simulink model "Control_model_10DOF_fin"  (R2016b)
settings: Solver=FixedStepAuto  StartTime=0.0  StopTime=10  FixedStep=0.0001  RelTol=1e-3
InitFcn:
  | Initialisation_ctr_10DOF_fin
values from neighbouring files (symbols this model uses):
  COM_Parameters = [-lpelvis/2;r2;0]    [Initialisation_ctr_10DOF_fin.m]
  DH_Parameters = [hfoot 0 ... (first row only)    [Initialisation_ctr_10DOF_fin.m]
  dTrunk = trunklbd(3)    [Initialisation_ctr_10DOF_fin.m]
  dxFootSM = dxFoot    [Initialisation_ctr_10DOF_fin.m]
  dxTrunk = 0.1    [Initialisation_ctr_10DOF_fin.m]
  Foot_Parameters = [0;-(lFoot/2-lHeel);0]    [Initialisation_ctr_10DOF_fin.m]
  HAA2HEE = [0; 0; 0.001]    [Initialisation_ctr_10DOF_fin.m]
  HEE2HFE = 0.5*[0.2; 0; 0]    [Initialisation_ctr_10DOF_fin.m]
  height_vrp = CoM_position(1)    [Initialisation_ctr_10DOF_fin.m]
  hTrunk = trunklbd(1)    [Initialisation_ctr_10DOF_fin.m]
  initial_CoM_position = R*CoM_position    [Initialisation_ctr_10DOF_fin.m]
  initial_CoM_velocity = [0;0;0]    [Initialisation_ctr_10DOF_fin.m]
  initial_left_foot = [0;0;-stance_width/2]    [Initialisation_ctr_10DOF_fin.m]
  initial_right_foot = [0;0;stance_width/2]    [Initialisation_ctr_10DOF_fin.m]
  initial_RorL = 0    [Initialisation_ctr_10DOF_fin.m]
  jointsinitial = [9;-15;6;0;0;6;-15;9]/180*pi    [Initialisation_ctr_10DOF_fin.m]
  K_DCM = 4.3*[1 0 0 ... (first row only)    [Initialisation_ctr_10DOF_fin.m]
  kD_left = mbody*[0.95 0 0 0 ... (first row only)    [Initialisation_ctr_10DOF_fin.m]
  kD_right = mbody*[0.12 0 0 0 ... (first row only)    [Initialisation_ctr_10DOF_fin.m]
  kI_left = mbody*[35 0 0 0 ... (first row only)    [Initialisation_ctr_10DOF_fin.m]
  kI_right = mbody*[38.2 0 0 0 ... (first row only)    [Initialisation_ctr_10DOF_fin.m]
  kP_left = mbody*[75 0 0 0 ... (first row only)    [Initialisation_ctr_10DOF_fin.m]
  kP_right = mbody*[5.6 0 0 0 ... (first row only)    [Initialisation_ctr_10DOF_fin.m]
  Lenght = [lShank;lThigh]    [Initialisation_ctr_10DOF_fin.m]
  lFootSM = lFoot    [Initialisation_ctr_10DOF_fin.m]
  lpelvis = wPelvis    [Initialisation_ctr_10DOF_fin.m]
  mass = mbody    (= 60)    [Initialisation_ctr_10DOF_fin.m]
  Masses = [mThigh; mShank; mTrunk]    [Initialisation_ctr_10DOF_fin.m]
  nb_step = 4    [Initialisation_ctr_10DOF_fin.m]
  nb_step_pattern = 20    [Initialisation_ctr_10DOF_fin.m]
  Pelvis_Parameters = [-lpelvis/2;hTrunk/2;0]    [Initialisation_ctr_10DOF_fin.m]
  stance_width = lpelvis    [Initialisation_ctr_10DOF_fin.m]
  stride_lenght = 0.50    (= 0.5)    [Initialisation_ctr_10DOF_fin.m]
  T_DS = time_DS    (= 0.4)    [Initialisation_ctr_10DOF_fin.m]
  T_IT = time_DS    (= 0.4)    [Initialisation_ctr_10DOF_fin.m]
  T_SS = time_swing    (= 1.6)    [Initialisation_ctr_10DOF_fin.m]
  time_DS = (time_stance-time_swing)/2    (= 0.4)    [Initialisation_ctr_10DOF_fin.m]
  time_stance = 60/100*time_stride    (= 2.4)    [Initialisation_ctr_10DOF_fin.m]
  time_step = time_stride/2    (= 2)    [Initialisation_ctr_10DOF_fin.m]
  time_swing = 40/100*time_stride    (= 1.6)    [Initialisation_ctr_10DOF_fin.m]
  validity_angle = [-20*pi/180 20*pi/180 ... (first row only)    [Initialisation_ctr_10DOF_fin.m]
  wTrunk = trunklbd(2)    [Initialisation_ctr_10DOF_fin.m]
  x4CoM = CoM_position(1)-XR4(1)    [Initialisation_ctr_10DOF_fin.m]
undefined symbols (not defined in the file or in its folder): dsegment, hFoot, l, lFoot, omega0_x, omega0_z, rho, wPelvis, X, Xp_x, Xp_z, Y, Z
undefined symbols (not defined in the file): k_grf, lShankSM, lThighSM, mShank, mThigh
libraries: nesl_utility x247, sm_lib x215, dspindex x12, FootPlacementLibrary x8, dspsigops x4, dspswit3 x1
(part 3 of 18)

== system Control_model_10DOF_fin/10DoF Walker SimMechanics Model/Hip FE ==
  torque : Inport
  Conv8 : nesl_utility/PS-Simulink Converter  PhysicalDomain=network_engine_domain  SubClassName=ps_output  LeftPortType=input  RightPortType=output  PseudoPeriodic=off  Frequencies=[]  Unit=rad  AffineConversion=off
  Conv9 : nesl_utility/PS-Simulink Converter  PhysicalDomain=network_engine_domain  SubClassName=ps_output  LeftPortType=input  RightPortType=output  PseudoPeriodic=off  Frequencies=[]  Unit=rad/s  AffineConversion=off
  Hip Joint : sm_lib/Joints/Revolute Joint  SenseConstraintForce=off  SenseConstraintForceX=off  SenseConstraintForceY=off  SenseConstraintForceZ=off  SenseConstraintTorque=off  SenseConstraintTorqueX=off  SenseConstraintTorqueY=off  SenseConstraintTorqueZ=off  SenseTotalForce=off  SenseTotalForceX=off  SenseTotalForceY=off  SenseTotalForceZ=off  SenseTotalTorque=off  SenseTotalTorqueX=off  SenseTotalTorqueY=off  SenseTotalTorqueZ=off  CompositeWrenchDir=FollowerOnBase  CompositeWrenchFrame=BaseFrame  EquilibriumPosition=0  EquilibriumPositionUnits=deg  SpringStiffness=0  SpringStiffnessUnits=N*m/deg  DampingCoefficient=joint_damping  DampingCoefficientUnits=N*m/(rad/s)  TorqueActuationMode=InputTorque  MotionActuationMode=ComputedMotion  SensePosition=on  SenseVelocity=on  SenseAcceleration=off  SenseTorqueForce=off  PositionTargetSpecify=on  PositionTargetPriority=High  PositionTargetValue=jointsinitial(3)  PositionTargetValueUnits=rad  VelocityTargetSpecify=off  VelocityTargetPriority=High  VelocityTargetValue=0  VelocityTargetValueUnits=deg/s
  MATLAB Function : MATLAB Function  TreatAsAtomicUnit=on
  Simulink-PS Converter7 : nesl_utility/Simulink-PS Converter  PhysicalDomain=network_engine_domain  SubClassName=ps_input  LeftPortType=input  RightPortType=output  PseudoPeriodic=off  Frequencies=[]  NoiseDistribution=none  NoiseParameters=[]  Unit=N*m  AffineConversion=off  InputFiltering=off  SimscapeFilterOrder=1  InputFilterTimeConstant=0.001  UdotUserProvided=1
  Conn1 : PMIOPort  Port=1  Side=Left
  Conn2 : PMIOPort  Port=2  Side=Right
  position : Outport
  velocity : Outport  Port=2
  wires:
  Conv8/1 -> MATLAB Function/1(joint), position/1
  Conv9/1 -> MATLAB Function/2(velocity), velocity/1
  MATLAB Function/1(torque) -> Simulink-PS Converter7/1
  torque/1 -> MATLAB Function/3(desired_torque)
  connections:
  Hip Joint/LConn1 -- Conn2/RConn1
  Hip Joint/LConn2 -- Simulink-PS Converter7/RConn1
  Hip Joint/RConn1 -- Conn1/RConn1
  Conv8/LConn1 -- Hip Joint/RConn2
  Hip Joint/RConn3 -- Conv9/LConn1

== system Control_model_10DOF_fin/10DoF Walker SimMechanics Model/Hip FE1 ==
  torque : Inport
  Conv8 : nesl_utility/PS-Simulink Converter  PhysicalDomain=network_engine_domain  SubClassName=ps_output  LeftPortType=input  RightPortType=output  PseudoPeriodic=off  Frequencies=[]  Unit=rad  AffineConversion=off
  Conv9 : nesl_utility/PS-Simulink Converter  PhysicalDomain=network_engine_domain  SubClassName=ps_output  LeftPortType=input  RightPortType=output  PseudoPeriodic=off  Frequencies=[]  Unit=rad/s  AffineConversion=off
  Hip Joint1 : sm_lib/Joints/Revolute Joint  SenseConstraintForce=off  SenseConstraintForceX=off  SenseConstraintForceY=off  SenseConstraintForceZ=off  SenseConstraintTorque=off  SenseConstraintTorqueX=off  SenseConstraintTorqueY=off  SenseConstraintTorqueZ=off  SenseTotalForce=off  SenseTotalForceX=off  SenseTotalForceY=off  SenseTotalForceZ=off  SenseTotalTorque=off  SenseTotalTorqueX=off  SenseTotalTorqueY=off  SenseTotalTorqueZ=off  CompositeWrenchDir=FollowerOnBase  CompositeWrenchFrame=BaseFrame  EquilibriumPosition=0  EquilibriumPositionUnits=deg  SpringStiffness=0  SpringStiffnessUnits=N*m/deg  DampingCoefficient=joint_damping  DampingCoefficientUnits=N*m/(rad/s)  TorqueActuationMode=InputTorque  MotionActuationMode=ComputedMotion  SensePosition=on  SenseVelocity=on  SenseAcceleration=off  SenseTorqueForce=off  PositionTargetSpecify=on  PositionTargetPriority=High  PositionTargetValue=jointsinitial(6)  PositionTargetValueUnits=rad  VelocityTargetSpecify=off  VelocityTargetPriority=High  VelocityTargetValue=0  VelocityTargetValueUnits=deg/s
  MATLAB Function : MATLAB Function  TreatAsAtomicUnit=on
  Simulink-PS Converter7 : nesl_utility/Simulink-PS Converter  PhysicalDomain=network_engine_domain  SubClassName=ps_input  LeftPortType=input  RightPortType=output  PseudoPeriodic=off  Frequencies=[]  NoiseDistribution=none  NoiseParameters=[]  Unit=N*m  AffineConversion=off  InputFiltering=off  SimscapeFilterOrder=1  InputFilterTimeConstant=0.001  UdotUserProvided=1
  Conn1 : PMIOPort  Port=1  Side=Left
  Conn2 : PMIOPort  Port=2  Side=Right
  position : Outport
  velocity : Outport  Port=2
  wires:
  Conv8/1 -> MATLAB Function/1(joint), position/1
  Conv9/1 -> MATLAB Function/2(velocity), velocity/1
  MATLAB Function/1(torque) -> Simulink-PS Converter7/1
  torque/1 -> MATLAB Function/3(desired_torque)
  connections:
  Hip Joint1/LConn1 -- Conn2/RConn1
  Simulink-PS Converter7/RConn1 -- Hip Joint1/LConn2
  Hip Joint1/RConn1 -- Conn1/RConn1
  Conv8/LConn1 -- Hip Joint1/RConn2
  Hip Joint1/RConn3 -- Conv9/LConn1

== system Control_model_10DOF_fin/10DoF Walker SimMechanics Model/Knee FE ==
  torque : Inport
  Conv8 : nesl_utility/PS-Simulink Converter  PhysicalDomain=network_engine_domain  SubClassName=ps_output  LeftPortType=input  RightPortType=output  PseudoPeriodic=off  Frequencies=[]  Unit=rad  AffineConversion=off
  Conv9 : nesl_utility/PS-Simulink Converter  PhysicalDomain=network_engine_domain  SubClassName=ps_output  LeftPortType=input  RightPortType=output  PseudoPeriodic=off  Frequencies=[]  Unit=rad/s  AffineConversion=off
  Knee Joint : sm_lib/Joints/Revolute Joint  SenseConstraintForce=off  SenseConstraintForceX=off  SenseConstraintForceY=off  SenseConstraintForceZ=off  SenseConstraintTorque=off  SenseConstraintTorqueX=off  SenseConstraintTorqueY=off  SenseConstraintTorqueZ=off  SenseTotalForce=off  SenseTotalForceX=off  SenseTotalForceY=off  SenseTotalForceZ=off  SenseTotalTorque=off  SenseTotalTorqueX=off  SenseTotalTorqueY=off  SenseTotalTorqueZ=off  CompositeWrenchDir=FollowerOnBase  CompositeWrenchFrame=BaseFrame  EquilibriumPosition=0  EquilibriumPositionUnits=deg  SpringStiffness=0  SpringStiffnessUnits=N*m/deg  DampingCoefficient=joint_damping  DampingCoefficientUnits=N*m/(rad/s)  TorqueActuationMode=InputTorque  MotionActuationMode=ComputedMotion  SensePosition=on  SenseVelocity=on  SenseAcceleration=off  SenseTorqueForce=off  PositionTargetSpecify=on  PositionTargetPriority=High  PositionTargetValue=jointsinitial(2)  PositionTargetValueUnits=rad  VelocityTargetSpecify=off  VelocityTargetPriority=High  VelocityTargetValue=0  VelocityTargetValueUnits=deg/s
  MATLAB Function : MATLAB Function  TreatAsAtomicUnit=on
  Simulink-PS Converter7 : nesl_utility/Simulink-PS Converter  PhysicalDomain=network_engine_domain  SubClassName=ps_input  LeftPortType=input  RightPortType=output  PseudoPeriodic=off  Frequencies=[]  NoiseDistribution=none  NoiseParameters=[]  Unit=N*m  AffineConversion=off  InputFiltering=off  SimscapeFilterOrder=1  InputFilterTimeConstant=0.001  UdotUserProvided=1
  Conn1 : PMIOPort  Port=1  Side=Left
  Conn2 : PMIOPort  Port=2  Side=Right
  position : Outport
  velocity : Outport  Port=2
  wires:
  Conv8/1 -> MATLAB Function/1(joint), position/1
  Conv9/1 -> MATLAB Function/2(velocity), velocity/1
  MATLAB Function/1(torque) -> Simulink-PS Converter7/1
  torque/1 -> MATLAB Function/3(desired_torque)
  connections:
  Knee Joint/LConn1 -- Conn2/RConn1
  Knee Joint/LConn2 -- Simulink-PS Converter7/RConn1
  Knee Joint/RConn1 -- Conn1/RConn1
  Knee Joint/RConn2 -- Conv8/LConn1
  Knee Joint/RConn3 -- Conv9/LConn1

== system Control_model_10DOF_fin/10DoF Walker SimMechanics Model/Knee FE1 ==
  torque : Inport
  Conv8 : nesl_utility/PS-Simulink Converter  PhysicalDomain=network_engine_domain  SubClassName=ps_output  LeftPortType=input  RightPortType=output  PseudoPeriodic=off  Frequencies=[]  Unit=rad  AffineConversion=off
  Conv9 : nesl_utility/PS-Simulink Converter  PhysicalDomain=network_engine_domain  SubClassName=ps_output  LeftPortType=input  RightPortType=output  PseudoPeriodic=off  Frequencies=[]  Unit=rad/s  AffineConversion=off
  Knee Joint1 : sm_lib/Joints/Revolute Joint  SenseConstraintForce=off  SenseConstraintForceX=off  SenseConstraintForceY=off  SenseConstraintForceZ=off  SenseConstraintTorque=off  SenseConstraintTorqueX=off  SenseConstraintTorqueY=off  SenseConstraintTorqueZ=off  SenseTotalForce=off  SenseTotalForceX=off  SenseTotalForceY=off  SenseTotalForceZ=off  SenseTotalTorque=off  SenseTotalTorqueX=off  SenseTotalTorqueY=off  SenseTotalTorqueZ=off  CompositeWrenchDir=FollowerOnBase  CompositeWrenchFrame=BaseFrame  EquilibriumPosition=0  EquilibriumPositionUnits=deg  SpringStiffness=0  SpringStiffnessUnits=N*m/deg  DampingCoefficient=joint_damping  DampingCoefficientUnits=N*m/(rad/s)  TorqueActuationMode=InputTorque  MotionActuationMode=ComputedMotion  SensePosition=on  SenseVelocity=on  SenseAcceleration=off  SenseTorqueForce=off  PositionTargetSpecify=on  PositionTargetPriority=High  PositionTargetValue=jointsinitial(7)  PositionTargetValueUnits=rad  VelocityTargetSpecify=off  VelocityTargetPriority=High  VelocityTargetValue=0  VelocityTargetValueUnits=deg/s
  MATLAB Function : MATLAB Function  TreatAsAtomicUnit=on
  Simulink-PS Converter7 : nesl_utility/Simulink-PS Converter  PhysicalDomain=network_engine_domain  SubClassName=ps_input  LeftPortType=input  RightPortType=output  PseudoPeriodic=off  Frequencies=[]  NoiseDistribution=none  NoiseParameters=[]  Unit=N*m  AffineConversion=off  InputFiltering=off  SimscapeFilterOrder=1  InputFilterTimeConstant=0.001  UdotUserProvided=1
  Conn1 : PMIOPort  Port=1  Side=Left
  Conn2 : PMIOPort  Port=2  Side=Right
  position : Outport
  velocity : Outport  Port=2
  wires:
  Conv8/1 -> MATLAB Function/1(joint), position/1
  Conv9/1 -> MATLAB Function/2(velocity), velocity/1
  MATLAB Function/1(torque) -> Simulink-PS Converter7/1
  torque/1 -> MATLAB Function/3(desired_torque)
  connections:
  Knee Joint1/LConn1 -- Conn2/RConn1
  Knee Joint1/LConn2 -- Simulink-PS Converter7/RConn1
  Knee Joint1/RConn1 -- Conn1/RConn1
  Knee Joint1/RConn2 -- Conv8/LConn1
  Knee Joint1/RConn3 -- Conv9/LConn1

== system Control_model_10DOF_fin/10DoF Walker SimMechanics Model/Scope x1 ==
  Input : Inport
  Demux : Demux  Outputs=3
  Scope1 : Scope
  Scope2 : Scope
  Scope3 : Scope
  wires:
  Input/1 -> Demux/1
  Demux/2 -> Scope1/1
  Demux/3 -> Scope2/1
  Demux/1 -> Scope3/1

== system Control_model_10DOF_fin/10DoF Walker SimMechanics Model/Shank ==
  Rigid  Transform : sm_lib/Frames and Transforms/Rigid Transform  TranslationMethod=StandardAxis  TranslationStandardOffset=l/2  TranslationLengthUnit=m  TranslationStandardAxis=+Y  TranslationCartesianOffset=[0 0 0]  TranslationROffset=0  TranslationROffsetUnits=m  TranslationZOffset=0  TranslationZOffsetUnits=m  TranslationThetaOffset=0  TranslationThetaOffsetUnits=deg  RotationMethod=StandardAxis  RotationAngleUnits=deg  RotationStandardAxis=+X  RotationAngle=-90  RotationArbitraryAxis=[0 0 1]  FollAlignAxisA=+X  BaseAlignAxisA=+Y  FollAlignAxisB=+Y  BaseAlignAxisB=+Z  RotationSequenceAxes=FollowerAxes  RotationSequence=XYX  RotationSequenceAngles=[0 0 0]  RotationSequenceAnglesUnits=deg  RotationMatrix=[1 0 0; 0 1 0; 0 0 1]
  Rigid  Transform1 : sm_lib/Frames and Transforms/Rigid Transform  TranslationMethod=Cartesian  TranslationStandardOffset=0  TranslationLengthUnit=m  TranslationStandardAxis=+Z  TranslationCartesianOffset=[ 0 0 l/2]  TranslationROffset=0  TranslationROffsetUnits=m  TranslationZOffset=0  TranslationZOffsetUnits=m  TranslationThetaOffset=0  TranslationThetaOffsetUnits=deg  RotationMethod=StandardAxis  RotationAngleUnits=deg  RotationStandardAxis=+X  RotationAngle=90  RotationArbitraryAxis=[0 0 1]  FollAlignAxisA=+X  BaseAlignAxisA=+Y  FollAlignAxisB=+Y  BaseAlignAxisB=+Z  RotationSequenceAxes=FollowerAxes  RotationSequence=XYX  RotationSequenceAngles=[0 0 0]  RotationSequenceAnglesUnits=deg  RotationMatrix=[1 0 0; 0 1 0; 0 0 1]
  Solid1 : sm_lib/Body Elements/Solid  InertiaType=CalculateFromGeometry  Mass=1  MassUnits=kg  CenterOfMass=[0 0 0]  CenterOfMassUnits=m  MomentsOfInertia=[1 1 1]  MomentsOfInertiaUnits=kg*m^2  ProductsOfInertia=[0 0 0]  ProductsOfInertiaUnits=kg*m^2  DensityBased=on  Density=rho  DensityUnits=kg/(m^3)  DoExposeReferenceFrame=on  SerializedFrames=<Frames/>  GraphicType=FromGeometry  MarkerShape=Sphere  MarkerSize=10  MarkerSizeUnits=m  GraphicVisPropType=AdvancedVisualProperties  GraphicDiffuseColor=[0 1 0]  GraphicSpecularColor=[0.5 0.5 0.5 1.0]  GraphicAmbientColor=[0.15 0.15 0.15 1.0]  GraphicEmissiveColor=[0.0 0.0 0.0 1.0]  GraphicShininess=75  GraphicOpacity=1.0  GeometryShape=Cylinder  RectangleSize=[1 1]  RectangleSizeUnits=m  BrickDimensions=[dsegment l dsegment]  BrickDimensionUnits=m  CylinderRadius=sqrt(m/(pi*rho*l))  CylinderRadiusUnits=m  CylinderLength=l  CylinderLengthUnits=m  SphereRadius=1  SphereRadiusUnits=m  EllipsoidRadii=[1 1 1]  EllipsoidRadiiUnits=m  ExtrusionCrossSection=[1 1; -1 1; -1 -1; 1 -1]  ExtrusionCrossSectionUnits=m  ExtrusionLength=1  ExtrusionLengthUnits=m  PolygonNumSides=3  PolygonOuterRadius=1  PolygonOuterRadiusUnits=m  ExtGeomFileType=STEP  ExtGeomFileUnits=m  RevolutionCrossSection=[1 1; 1 -1; 2 -1; 2 1]  RevolutionCrossSectionUnits=m  RevolutionExtent=Full  RevolutionAngle=180  RevolutionAngleUnits=deg
  Ankle : PMIOPort  Port=1  Side=Left
  Knee : PMIOPort  Port=2  Side=Right
  connections:
  Rigid  Transform/LConn1 -- Ankle/RConn1
  Rigid  Transform1/RConn1 -- Knee/RConn1
  Solid1/RConn1 -- Rigid  Transform1/LConn1 -- Rigid  Transform/RConn1

== system Control_model_10DOF_fin/10DoF Walker SimMechanics Model/Shank1 ==
  Rigid  Transform : sm_lib/Frames and Transforms/Rigid Transform  TranslationMethod=StandardAxis  TranslationStandardOffset=l/2  TranslationLengthUnit=m  TranslationStandardAxis=+Y  TranslationCartesianOffset=[0 0 0]  TranslationROffset=0  TranslationROffsetUnits=m  TranslationZOffset=0  TranslationZOffsetUnits=m  TranslationThetaOffset=0  TranslationThetaOffsetUnits=deg  RotationMethod=StandardAxis  RotationAngleUnits=deg  RotationStandardAxis=+X  RotationAngle=-90  RotationArbitraryAxis=[0 0 1]  FollAlignAxisA=+X  BaseAlignAxisA=+Y  FollAlignAxisB=+Y  BaseAlignAxisB=+Z  RotationSequenceAxes=FollowerAxes  RotationSequence=XYX  RotationSequenceAngles=[0 0 0]  RotationSequenceAnglesUnits=deg  RotationMatrix=[1 0 0; 0 1 0; 0 0 1]
  Rigid  Transform1 : sm_lib/Frames and Transforms/Rigid Transform  TranslationMethod=Cartesian  TranslationStandardOffset=0  TranslationLengthUnit=m  TranslationStandardAxis=+Z  TranslationCartesianOffset=[ 0 0 l/2]  TranslationROffset=0  TranslationROffsetUnits=m  TranslationZOffset=0  TranslationZOffsetUnits=m  TranslationThetaOffset=0  TranslationThetaOffsetUnits=deg  RotationMethod=StandardAxis  RotationAngleUnits=deg  RotationStandardAxis=+X  RotationAngle=90  RotationArbitraryAxis=[0 0 1]  FollAlignAxisA=+X  BaseAlignAxisA=+Y  FollAlignAxisB=+Y  BaseAlignAxisB=+Z  RotationSequenceAxes=FollowerAxes  RotationSequence=XYX  RotationSequenceAngles=[0 0 0]  RotationSequenceAnglesUnits=deg  RotationMatrix=[1 0 0; 0 1 0; 0 0 1]
  Solid1 : sm_lib/Body Elements/Solid  InertiaType=CalculateFromGeometry  Mass=1  MassUnits=kg  CenterOfMass=[0 0 0]  CenterOfMassUnits=m  MomentsOfInertia=[1 1 1]  MomentsOfInertiaUnits=kg*m^2  ProductsOfInertia=[0 0 0]  ProductsOfInertiaUnits=kg*m^2  DensityBased=on  Density=rho  DensityUnits=kg/(m^3)  DoExposeReferenceFrame=on  SerializedFrames=<Frames/>  GraphicType=FromGeometry  MarkerShape=Sphere  MarkerSize=10  MarkerSizeUnits=m  GraphicVisPropType=AdvancedVisualProperties  GraphicDiffuseColor=[0 1 0]  GraphicSpecularColor=[0.5 0.5 0.5 1.0]  GraphicAmbientColor=[0.15 0.15 0.15 1.0]  GraphicEmissiveColor=[0.0 0.0 0.0 1.0]  GraphicShininess=75  GraphicOpacity=1.0  GeometryShape=Cylinder  RectangleSize=[1 1]  RectangleSizeUnits=m  BrickDimensions=[dsegment l dsegment]  BrickDimensionUnits=m  CylinderRadius=sqrt(m/(pi*rho*l))  CylinderRadiusUnits=m  CylinderLength=l  CylinderLengthUnits=m  SphereRadius=1  SphereRadiusUnits=m  EllipsoidRadii=[1 1 1]  EllipsoidRadiiUnits=m  ExtrusionCrossSection=[1 1; -1 1; -1 -1; 1 -1]  ExtrusionCrossSectionUnits=m  ExtrusionLength=1  ExtrusionLengthUnits=m  PolygonNumSides=3  PolygonOuterRadius=1  PolygonOuterRadiusUnits=m  ExtGeomFileType=STEP  ExtGeomFileUnits=m  RevolutionCrossSection=[1 1; 1 -1; 2 -1; 2 1]  RevolutionCrossSectionUnits=m  RevolutionExtent=Full  RevolutionAngle=180  RevolutionAngleUnits=deg
  Ankle : PMIOPort  Port=1  Side=Left
  Knee : PMIOPort  Port=2  Side=Right
  connections:
  Rigid  Transform/RConn1 -- Rigid  Transform1/LConn1 -- Solid1/RConn1
  Rigid  Transform1/RConn1 -- Knee/RConn1
  Rigid  Transform/LConn1 -- Ankle/RConn1

== system Control_model_10DOF_fin/10DoF Walker SimMechanics Model/Thigh1 ==
  Rigid  Transform : sm_lib/Frames and Transforms/Rigid Transform  TranslationMethod=Cartesian  TranslationStandardOffset=0  TranslationLengthUnit=m  TranslationStandardAxis=+Z  TranslationCartesianOffset=[0 l/2 0]  TranslationROffset=0  TranslationROffsetUnits=m  TranslationZOffset=0  TranslationZOffsetUnits=m  TranslationThetaOffset=0  TranslationThetaOffsetUnits=deg  RotationMethod=StandardAxis  RotationAngleUnits=deg  RotationStandardAxis=+X  RotationAngle=-90  RotationArbitraryAxis=[0 0 1]  FollAlignAxisA=+X  BaseAlignAxisA=+Y  FollAlignAxisB=+Y  BaseAlignAxisB=+Z  RotationSequenceAxes=FollowerAxes  RotationSequence=XYX  RotationSequenceAngles=[0 0 0]  RotationSequenceAnglesUnits=deg  RotationMatrix=[1 0 0; 0 1 0; 0 0 1]
  Rigid  Transform1 : sm_lib/Frames and Transforms/Rigid Transform  TranslationMethod=Cartesian  TranslationStandardOffset=0  TranslationLengthUnit=m  TranslationStandardAxis=+Z  TranslationCartesianOffset=[0 0 l/2]  TranslationROffset=0  TranslationROffsetUnits=m  TranslationZOffset=0  TranslationZOffsetUnits=m  TranslationThetaOffset=0  TranslationThetaOffsetUnits=deg  RotationMethod=StandardAxis  RotationAngleUnits=deg  RotationStandardAxis=+X  RotationAngle=90  RotationArbitraryAxis=[0 0 1]  FollAlignAxisA=+X  BaseAlignAxisA=+Y  FollAlignAxisB=+Y  BaseAlignAxisB=+Z  RotationSequenceAxes=FollowerAxes  RotationSequence=XYX  RotationSequenceAngles=[0 0 0]  RotationSequenceAnglesUnits=deg  RotationMatrix=[1 0 0; 0 1 0; 0 0 1]
  Solid : sm_lib/Body Elements/Solid  InertiaType=CalculateFromGeometry  Mass=1  MassUnits=kg  CenterOfMass=[0 0 0]  CenterOfMassUnits=m  MomentsOfInertia=[1 1 1]  MomentsOfInertiaUnits=kg*m^2  ProductsOfInertia=[0 0 0]  ProductsOfInertiaUnits=kg*m^2  DensityBased=on  Density=rho  DensityUnits=kg/(m^3)  DoExposeReferenceFrame=on  SerializedFrames=<Frames/>  GraphicType=FromGeometry  MarkerShape=Sphere  MarkerSize=10  MarkerSizeUnits=m  GraphicVisPropType=AdvancedVisualProperties  GraphicDiffuseColor=[0 1 0]  GraphicSpecularColor=[0.5 0.5 0.5 1.0]  GraphicAmbientColor=[0.15 0.15 0.15 1.0]  GraphicEmissiveColor=[0.0 0.0 0.0 1.0]  GraphicShininess=75  GraphicOpacity=1.0  GeometryShape=Cylinder  RectangleSize=[1 1]  RectangleSizeUnits=m  BrickDimensions=[dsegment l dsegment]  BrickDimensionUnits=m  CylinderRadius=sqrt(m/(pi*rho*l))  CylinderRadiusUnits=m  CylinderLength=l  CylinderLengthUnits=m  SphereRadius=1  SphereRadiusUnits=m  EllipsoidRadii=[1 1 1]  EllipsoidRadiiUnits=m  ExtrusionCrossSection=[1 1; -1 1; -1 -1; 1 -1]  ExtrusionCrossSectionUnits=m  ExtrusionLength=1  ExtrusionLengthUnits=m  PolygonNumSides=3  PolygonOuterRadius=1  PolygonOuterRadiusUnits=m  ExtGeomFileType=STEP  ExtGeomFileUnits=m  RevolutionCrossSection=[1 1; 1 -1; 2 -1; 2 1]  RevolutionCrossSectionUnits=m  RevolutionExtent=Full  RevolutionAngle=180  RevolutionAngleUnits=deg
  Knee : PMIOPort  Port=1  Side=Left
  Hip : PMIOPort  Port=2  Side=Right
  connections:
  Rigid  Transform/LConn1 -- Knee/RConn1
  Rigid  Transform1/LConn1 -- Solid/RConn1 -- Rigid  Transform/RConn1
  Rigid  Transform1/RConn1 -- Hip/RConn1

== system Control_model_10DOF_fin/10DoF Walker SimMechanics Model/Thigh2 ==
  Rigid  Transform : sm_lib/Frames and Transforms/Rigid Transform  TranslationMethod=Cartesian  TranslationStandardOffset=0  TranslationLengthUnit=m  TranslationStandardAxis=+Z  TranslationCartesianOffset=[0 l/2 0]  TranslationROffset=0  TranslationROffsetUnits=m  TranslationZOffset=0  TranslationZOffsetUnits=m  TranslationThetaOffset=0  TranslationThetaOffsetUnits=deg  RotationMethod=StandardAxis  RotationAngleUnits=deg  RotationStandardAxis=+X  RotationAngle=-90  RotationArbitraryAxis=[0 0 1]  FollAlignAxisA=+X  BaseAlignAxisA=+Y  FollAlignAxisB=+Y  BaseAlignAxisB=+Z  RotationSequenceAxes=FollowerAxes  RotationSequence=XYX  RotationSequenceAngles=[0 0 0]  RotationSequenceAnglesUnits=deg  RotationMatrix=[1 0 0; 0 1 0; 0 0 1]
  Rigid  Transform1 : sm_lib/Frames and Transforms/Rigid Transform  TranslationMethod=Cartesian  TranslationStandardOffset=0  TranslationLengthUnit=m  TranslationStandardAxis=+Z  TranslationCartesianOffset=[0 0 l/2]  TranslationROffset=0  TranslationROffsetUnits=m  TranslationZOffset=0  TranslationZOffsetUnits=m  TranslationThetaOffset=0  TranslationThetaOffsetUnits=deg  RotationMethod=StandardAxis  RotationAngleUnits=deg  RotationStandardAxis=+X  RotationAngle=90  RotationArbitraryAxis=[0 0 1]  FollAlignAxisA=+X  BaseAlignAxisA=+Y  FollAlignAxisB=+Y  BaseAlignAxisB=+Z  RotationSequenceAxes=FollowerAxes  RotationSequence=XYX  RotationSequenceAngles=[0 0 0]  RotationSequenceAnglesUnits=deg  RotationMatrix=[1 0 0; 0 1 0; 0 0 1]
  Solid : sm_lib/Body Elements/Solid  InertiaType=CalculateFromGeometry  Mass=1  MassUnits=kg  CenterOfMass=[0 0 0]  CenterOfMassUnits=m  MomentsOfInertia=[1 1 1]  MomentsOfInertiaUnits=kg*m^2  ProductsOfInertia=[0 0 0]  ProductsOfInertiaUnits=kg*m^2  DensityBased=on  Density=rho  DensityUnits=kg/(m^3)  DoExposeReferenceFrame=on  SerializedFrames=<Frames/>  GraphicType=FromGeometry  MarkerShape=Sphere  MarkerSize=10  MarkerSizeUnits=m  GraphicVisPropType=AdvancedVisualProperties  GraphicDiffuseColor=[0 1 0]  GraphicSpecularColor=[0.5 0.5 0.5 1.0]  GraphicAmbientColor=[0.15 0.15 0.15 1.0]  GraphicEmissiveColor=[0.0 0.0 0.0 1.0]  GraphicShininess=75  GraphicOpacity=1.0  GeometryShape=Cylinder  RectangleSize=[1 1]  RectangleSizeUnits=m  BrickDimensions=[dsegment l dsegment]  BrickDimensionUnits=m  CylinderRadius=sqrt(m/(pi*rho*l))  CylinderRadiusUnits=m  CylinderLength=l  CylinderLengthUnits=m  SphereRadius=1  SphereRadiusUnits=m  EllipsoidRadii=[1 1 1]  EllipsoidRadiiUnits=m  ExtrusionCrossSection=[1 1; -1 1; -1 -1; 1 -1]  ExtrusionCrossSectionUnits=m  ExtrusionLength=1  ExtrusionLengthUnits=m  PolygonNumSides=3  PolygonOuterRadius=1  PolygonOuterRadiusUnits=m  ExtGeomFileType=STEP  ExtGeomFileUnits=m  RevolutionCrossSection=[1 1; 1 -1; 2 -1; 2 1]  RevolutionCrossSectionUnits=m  RevolutionExtent=Full  RevolutionAngle=180  RevolutionAngleUnits=deg
  Knee : PMIOPort  Port=1  Side=Left
  Hip : PMIOPort  Port=2  Side=Right
  connections:
  Rigid  Transform1/RConn1 -- Hip/RConn1
  Solid/RConn1 -- Rigid  Transform1/LConn1 -- Rigid  Transform/RConn1
  Rigid  Transform/LConn1 -- Knee/RConn1

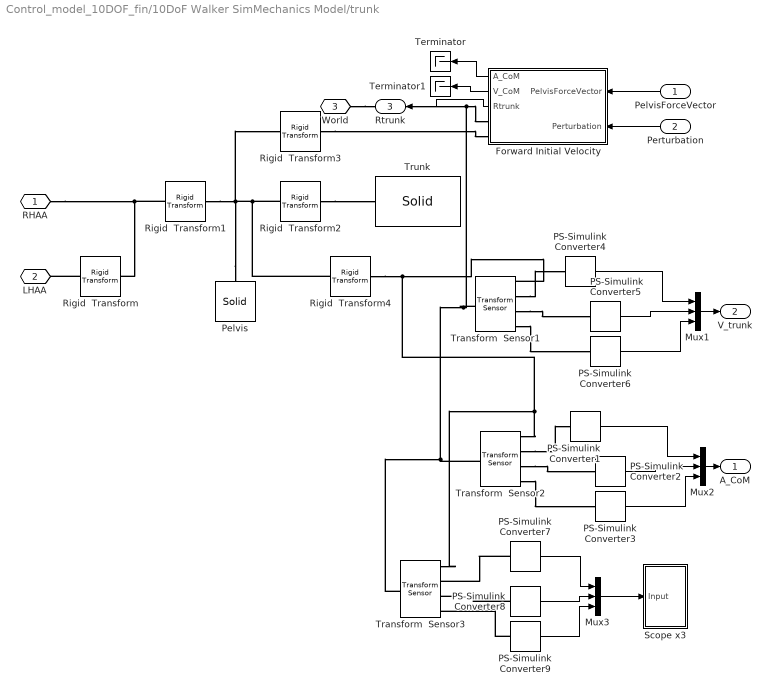
== system Control_model_10DOF_fin/10DoF Walker SimMechanics Model/trunk ==
  PelvisForceVector : Inport
  Perturbation : Inport  Port=2
  Forward Initial Velocity : Subsystem
  Mux1 : Mux  Inputs=3
  Mux2 : Mux  Inputs=3
  Mux3 : Mux  Inputs=3
  PS-Simulink Converter{1..9} (9 alike) : nesl_utility/PS-Simulink Converter  PhysicalDomain=network_engine_domain  SubClassName=ps_output  LeftPortType=input  RightPortType=output  PseudoPeriodic=off  Frequencies=[]  Unit=1  AffineConversion=off
  Pelvis : sm_lib/Body Elements/Solid  InertiaType=CalculateFromGeometry  Mass=1  MassUnits=kg  CenterOfMass=[0 0 0]  CenterOfMassUnits=m  MomentsOfInertia=[1 1 1]  MomentsOfInertiaUnits=kg*m^2  ProductsOfInertia=[0 0 0]  ProductsOfInertiaUnits=kg*m^2  DensityBased=on  Density=1000  DensityUnits=kg/(m^3)  DoExposeReferenceFrame=on  SerializedFrames=<Frames/>  GraphicType=FromGeometry  MarkerShape=Sphere  MarkerSize=10  MarkerSizeUnits=m  GraphicVisPropType=AdvancedVisualProperties  GraphicDiffuseColor=[0 0 1]  GraphicSpecularColor=[0.5 0.5 0.5 1.0]  GraphicAmbientColor=[0.15 0.15 0.15 1.0]  GraphicEmissiveColor=[0.0 0.0 0.0 1.0]  GraphicShininess=75  GraphicOpacity=1.0  GeometryShape=Brick  RectangleSize=[1 1]  RectangleSizeUnits=m  BrickDimensions=[wPelvis dsegment dsegment]  BrickDimensionUnits=m  CylinderRadius=1  CylinderRadiusUnits=m  CylinderLength=1  CylinderLengthUnits=m  SphereRadius=1  SphereRadiusUnits=m  EllipsoidRadii=[1 1 1]  EllipsoidRadiiUnits=m  ExtrusionCrossSection=[1 1; -1 1; -1 -1; 1 -1]  ExtrusionCrossSectionUnits=m  ExtrusionLength=1  ExtrusionLengthUnits=m  PolygonNumSides=3  PolygonOuterRadius=1  PolygonOuterRadiusUnits=m  ExtGeomFileType=STEP  ExtGeomFileUnits=m  RevolutionCrossSection=[1 1; 1 -1; 2 -1; 2 1]  RevolutionCrossSectionUnits=m  RevolutionExtent=Full  RevolutionAngle=180  RevolutionAngleUnits=deg
  Rigid  Transform : sm_lib/Frames and Transforms/Rigid Transform  TranslationMethod=Cartesian  TranslationStandardOffset=0  TranslationLengthUnit=m  TranslationStandardAxis=+Z  TranslationCartesianOffset=[wPelvis 0 0]  TranslationROffset=0  TranslationROffsetUnits=m  TranslationZOffset=0  TranslationZOffsetUnits=m  TranslationThetaOffset=0  TranslationThetaOffsetUnits=deg  RotationMethod=None  RotationAngleUnits=deg  RotationStandardAxis=+Z  RotationAngle=0  RotationArbitraryAxis=[0 0 1]  FollAlignAxisA=+X  BaseAlignAxisA=+Y  FollAlignAxisB=+Y  BaseAlignAxisB=+Z  RotationSequenceAxes=FollowerAxes  RotationSequence=XYX  RotationSequenceAngles=[0 0 0]  RotationSequenceAnglesUnits=deg  RotationMatrix=[1 0 0; 0 1 0; 0 0 1]
  Rigid  Transform1 : sm_lib/Frames and Transforms/Rigid Transform  TranslationMethod=StandardAxis  TranslationStandardOffset=wPelvis/2  TranslationLengthUnit=m  TranslationStandardAxis=+X  TranslationCartesianOffset=[0 0 0]  TranslationROffset=0  TranslationROffsetUnits=m  TranslationZOffset=0  TranslationZOffsetUnits=m  TranslationThetaOffset=0  TranslationThetaOffsetUnits=deg  RotationMethod=None  RotationAngleUnits=deg  RotationStandardAxis=+X  RotationAngle=0  RotationArbitraryAxis=[0 0 1]  FollAlignAxisA=+X  BaseAlignAxisA=+Y  FollAlignAxisB=+Y  BaseAlignAxisB=+Z  RotationSequenceAxes=FollowerAxes  RotationSequence=XYX  RotationSequenceAngles=[0 0 0]  RotationSequenceAnglesUnits=deg  RotationMatrix=[1 0 0; 0 1 0; 0 0 1]
  Rigid  Transform2 : sm_lib/Frames and Transforms/Rigid Transform  TranslationMethod=Cartesian  TranslationStandardOffset=0  TranslationLengthUnit=m  TranslationStandardAxis=+Z  TranslationCartesianOffset=[0 hTrunk/2 dxTrunk]  TranslationROffset=0  TranslationROffsetUnits=m  TranslationZOffset=0  TranslationZOffsetUnits=m  TranslationThetaOffset=0  TranslationThetaOffsetUnits=deg  RotationMethod=StandardAxis  RotationAngleUnits=deg  RotationStandardAxis=+Y  RotationAngle=180  RotationArbitraryAxis=[0 0 1]  FollAlignAxisA=+X  BaseAlignAxisA=+Y  FollAlignAxisB=+Y  BaseAlignAxisB=+Z  RotationSequenceAxes=FollowerAxes  RotationSequence=XYX  RotationSequenceAngles=[0 0 0]  RotationSequenceAnglesUnits=deg  RotationMatrix=[1 0 0; 0 1 0; 0 0 1]
  Rigid  Transform3 : sm_lib/Frames and Transforms/Rigid Transform  TranslationMethod=None  TranslationStandardOffset=0  TranslationLengthUnit=m  TranslationStandardAxis=+Z  TranslationCartesianOffset=[0 0 0]  TranslationROffset=0  TranslationROffsetUnits=m  TranslationZOffset=0  TranslationZOffsetUnits=m  TranslationThetaOffset=0  TranslationThetaOffsetUnits=deg  RotationMethod=StandardAxis  RotationAngleUnits=deg  RotationStandardAxis=+Y  RotationAngle=-90  RotationArbitraryAxis=[0 0 1]  FollAlignAxisA=+X  BaseAlignAxisA=+Y  FollAlignAxisB=+Y  BaseAlignAxisB=+Z  RotationSequenceAxes=FollowerAxes  RotationSequence=XYX  RotationSequenceAngles=[0 0 0]  RotationSequenceAnglesUnits=deg  RotationMatrix=[1 0 0; 0 1 0; 0 0 1]
  Rigid  Transform4 : sm_lib/Frames and Transforms/Rigid Transform  TranslationMethod=Cartesian  TranslationStandardOffset=0  TranslationLengthUnit=m  TranslationStandardAxis=+Z  TranslationCartesianOffset=[0 x4CoM dxTrunk]  TranslationROffset=0  TranslationROffsetUnits=m  TranslationZOffset=0  TranslationZOffsetUnits=m  TranslationThetaOffset=0  TranslationThetaOffsetUnits=deg  RotationMethod=StandardAxis  RotationAngleUnits=deg  RotationStandardAxis=+Y  RotationAngle=180  RotationArbitraryAxis=[0 0 1]  FollAlignAxisA=+X  BaseAlignAxisA=+Y  FollAlignAxisB=+Y  BaseAlignAxisB=+Z  RotationSequenceAxes=FollowerAxes  RotationSequence=XYX  RotationSequenceAngles=[0 0 0]  RotationSequenceAnglesUnits=deg  RotationMatrix=[1 0 0; 0 1 0; 0 0 1]
  Scope x3 : Subsystem
  Terminator : Terminator
  Terminator1 : Terminator
  Transform  Sensor1 : sm_lib/Frames and Transforms/Transform Sensor  MeasurementFrame=World  SenseAngle=off  SenseAxis=off  SenseAngle1=off  SenseAngle2=off  SenseAngle3=off  SenseQ=off  SenseR=off  SenseOmegaX=off  SenseOmegaY=off  SenseOmegaZ=off  SenseOmega1=off  SenseOmega2=off  SenseOmega3=off  SenseQDot=off  SenseRDot=off  SenseAlphaX=off  SenseAlphaY=off  SenseAlphaZ=off  SenseAlpha1=off  SenseAlpha2=off  SenseAlpha3=off  SenseQDDot=off  SenseRDDot=off  SenseX=off  SenseY=off  SenseZ=off  SenseRad=off  SenseAzim=off  SenseDist=off  SenseInc=off  SenseXDot=on  SenseYDot=on  SenseZDot=on  SenseRadDot=off  SenseAzimDot=off  SenseDistDot=off  SenseIncDot=off  SenseXDDot=off  SenseYDDot=off  SenseZDDot=off  SenseRadDDot=off  SenseAzimDDot=off  SenseDistDDot=off  SenseIncDDot=off
  Transform  Sensor2 : sm_lib/Frames and Transforms/Transform Sensor  MeasurementFrame=World  SenseAngle=off  SenseAxis=off  SenseAngle1=off  SenseAngle2=off  SenseAngle3=off  SenseQ=off  SenseR=off  SenseOmegaX=off  SenseOmegaY=off  SenseOmegaZ=off  SenseOmega1=off  SenseOmega2=off  SenseOmega3=off  SenseQDot=off  SenseRDot=off  SenseAlphaX=off  SenseAlphaY=off  SenseAlphaZ=off  SenseAlpha1=off  SenseAlpha2=off  SenseAlpha3=off  SenseQDDot=off  SenseRDDot=off  SenseX=off  SenseY=off  SenseZ=off  SenseRad=off  SenseAzim=off  SenseDist=off  SenseInc=off  SenseXDot=off  SenseYDot=off  SenseZDot=off  SenseRadDot=off  SenseAzimDot=off  SenseDistDot=off  SenseIncDot=off  SenseXDDot=on  SenseYDDot=on  SenseZDDot=on  SenseRadDDot=off  SenseAzimDDot=off  SenseDistDDot=off  SenseIncDDot=off
  Transform  Sensor3 : sm_lib/Frames and Transforms/Transform Sensor  MeasurementFrame=World  SenseAngle=off  SenseAxis=off  SenseAngle1=off  SenseAngle2=off  SenseAngle3=off  SenseQ=off  SenseR=off  SenseOmegaX=off  SenseOmegaY=off  SenseOmegaZ=off  SenseOmega1=off  SenseOmega2=off  SenseOmega3=off  SenseQDot=off  SenseRDot=off  SenseAlphaX=off  SenseAlphaY=off  SenseAlphaZ=off  SenseAlpha1=off  SenseAlpha2=off  SenseAlpha3=off  SenseQDDot=off  SenseRDDot=off  SenseX=on  SenseY=on  SenseZ=on  SenseRad=off  SenseAzim=off  SenseDist=off  SenseInc=off  SenseXDot=off  SenseYDot=off  SenseZDot=off  SenseRadDot=off  SenseAzimDot=off  SenseDistDot=off  SenseIncDot=off  SenseXDDot=off  SenseYDDot=off  SenseZDDot=off  SenseRadDDot=off  SenseAzimDDot=off  SenseDistDDot=off  SenseIncDDot=off
  Trunk : sm_lib/Body Elements/Solid  InertiaType=CalculateFromGeometry  Mass=1  MassUnits=kg  CenterOfMass=[0 0 0]  CenterOfMassUnits=m  MomentsOfInertia=[1 1 1]  MomentsOfInertiaUnits=kg*m^2  ProductsOfInertia=[0 0 0]  ProductsOfInertiaUnits=kg*m^2  DensityBased=on  Density=1000  DensityUnits=kg/(m^3)  DoExposeReferenceFrame=on  SerializedFrames=<Frames/>  GraphicType=FromGeometry  MarkerShape=Sphere  MarkerSize=10  MarkerSizeUnits=m  GraphicVisPropType=AdvancedVisualProperties  GraphicDiffuseColor=[0 0 1]  GraphicSpecularColor=[0.5 0.5 0.5 1.0]  GraphicAmbientColor=[0.15 0.15 0.15 1.0]  GraphicEmissiveColor=[0.0 0.0 0.0 1.0]  GraphicShininess=75  GraphicOpacity=1.0  GeometryShape=Brick  RectangleSize=[1 1]  RectangleSizeUnits=m  BrickDimensions=[wTrunk hTrunk dTrunk]  BrickDimensionUnits=m  CylinderRadius=1  CylinderRadiusUnits=m  CylinderLength=1  CylinderLengthUnits=m  SphereRadius=1  SphereRadiusUnits=m  EllipsoidRadii=[1 1 1]  EllipsoidRadiiUnits=m  ExtrusionCrossSection=[1 1; -1 1; -1 -1; 1 -1]  ExtrusionCrossSectionUnits=m  ExtrusionLength=1  ExtrusionLengthUnits=m  PolygonNumSides=3  PolygonOuterRadius=1  PolygonOuterRadiusUnits=m  ExtGeomFileType=STEP  ExtGeomFileUnits=m  RevolutionCrossSection=[1 1; 1 -1; 2 -1; 2 1]  RevolutionCrossSectionUnits=m  RevolutionExtent=Full  RevolutionAngle=180  RevolutionAngleUnits=deg
  RHAA : PMIOPort  Port=1  Side=Left
  LHAA : PMIOPort  Port=2  Side=Left
  World : PMIOPort  Port=3  Side=Right
  A_CoM : Outport
  V_trunk : Outport  Port=2
  Rtrunk : Outport  Port=3
  wires:
  PelvisForceVector/1 -> Forward Initial Velocity/1(PelvisForceVector)
  PS-Simulink Converter6/1 -> Mux1/3
  Mux1/1 -> V_trunk/1
  PS-Simulink Converter5/1 -> Mux1/2
  PS-Simulink Converter4/1 -> Mux1/1
  PS-Simulink Converter3/1 -> Mux2/3
  PS-Simulink Converter2/1 -> Mux2/2
  PS-Simulink Converter1/1 -> Mux2/1
  Mux2/1 -> A_CoM/1
  PS-Simulink Converter9/1 -> Mux3/3
  PS-Simulink Converter8/1 -> Mux3/2
  PS-Simulink Converter7/1 -> Mux3/1
  Mux3/1 -> Scope x3/1(Input)
  Forward Initial Velocity/3(Rtrunk) -> Rtrunk/1
  Perturbation/1 -> Forward Initial Velocity/2(Perturbation)
  Forward Initial Velocity/1(A_CoM) -> Terminator/1
  Forward Initial Velocity/2(V_CoM) -> Terminator1/1
  connections:
  RHAA/RConn1 -- Rigid  Transform1/LConn1 -- Rigid  Transform/LConn1
  Pelvis/RConn1 -- Rigid  Transform4/LConn1 -- Rigid  Transform2/LConn1 -- Rigid  Transform3/LConn1 -- Rigid  Transform1/RConn1
  Rigid  Transform/RConn1 -- LHAA/RConn1
  World/RConn1 -- Transform  Sensor3/LConn1 -- Transform  Sensor2/LConn1 -- Transform  Sensor1/LConn1 -- Forward Initial Velocity/RConn1
  Transform  Sensor1/RConn3 -- PS-Simulink Converter5/LConn1
  Transform  Sensor1/RConn4 -- PS-Simulink Converter6/LConn1
  Transform  Sensor1/RConn2 -- PS-Simulink Converter4/LConn1
  Transform  Sensor2/RConn4 -- PS-Simulink Converter3/LConn1
  Transform  Sensor2/RConn3 -- PS-Simulink Converter2/LConn1
  Transform  Sensor2/RConn2 -- PS-Simulink Converter1/LConn1
  Rigid  Transform2/RConn1 -- Trunk/RConn1
  PS-Simulink Converter9/LConn1 -- Transform  Sensor3/RConn4
  PS-Simulink Converter7/LConn1 -- Transform  Sensor3/RConn2
  PS-Simulink Converter8/LConn1 -- Transform  Sensor3/RConn3
  Rigid  Transform4/RConn1 -- Transform  Sensor3/RConn1 -- Transform  Sensor2/RConn1 -- Transform  Sensor1/RConn1
  Rigid  Transform3/RConn1 -- Forward Initial Velocity/RConn2

== system Control_model_10DOF_fin/Control/Double_Support ==
  RorL : Inport
  DCM_position : Inport  Port=2
  DCM_velocity : Inport  Port=3
  FK_info : Inport  Port=4
  joint_angle : Inport  Port=5
  joint_velocity : Inport  Port=6
  hip_trajectory : Inport  Port=7
  knee_trajectory : Inport  Port=8
  Action Port : ActionPort  ActionType=case
  Constant2 : Constant  Value=[0;0;0]
  If Right stance phase : If  IfExpression=u1 ==0
  Left stance phase1 : Subsystem
  Merge{1..4} (4 alike) : Merge
  Right stance phase : Subsystem
  Force : Outport
  Torques : Outport  Port=2
  r_vrp : Outport  Port=3
  r_extrapolated_CoM : Outport  Port=4
  Foot_adjust : Outport  Port=5
  wires:
  RorL/1 -> If Right stance phase/1
  If Right stance phase/1 -> Right stance phase/Action
  If Right stance phase/2 -> Left stance phase1/Action
  Merge4/1 -> Force/1
  Merge1/1 -> Torques/1
  Merge2/1 -> r_vrp/1
  Merge3/1 -> r_extrapolated_CoM/1
  Right stance phase/1(Force_des) -> Merge4/1
  Left stance phase1/1(Force_des) -> Merge4/2
  Right stance phase/2(Torques_des) -> Merge1/1
  Left stance phase1/2(Torques_des) -> Merge1/2
  Right stance phase/3(r_vrp) -> Merge2/1
  Left stance phase1/3(r_vrp) -> Merge2/2
  Right stance phase/4(r_extrapolated_CoM) -> Merge3/1
  Left stance phase1/4(r_extrapolated_CoM) -> Merge3/2
  DCM_position/1 -> Left stance phase1/1(DCM_position), Right stance phase/1(DCM_position)
  DCM_velocity/1 -> Left stance phase1/2(DCM_velocity), Right stance phase/2(DCM_velocity)
  FK_info/1 -> Right stance phase/3(FK_info), Left stance phase1/3(FK_info)
  joint_angle/1 -> Right stance phase/4(joint_angle), Left stance phase1/4(joint_angle)
  joint_velocity/1 -> Left stance phase1/5(joint_velocity), Right stance phase/5(joint_velocity)
  hip_trajectory/1 -> Left stance phase1/6(hip_trajectory), Right stance phase/6(hip_trajectory)
  Constant2/1 -> Foot_adjust/1
  knee_trajectory/1 -> Left stance phase1/7(knee_trajectory), Right stance phase/7(knee_trajectory)

== system Control_model_10DOF_fin/Control/Finish_Swing_Phase ==
  RorL : Inport  OutDataTypeStr=boolean  PortDimensions=1
  DCM_position : Inport  Port=2
  DCM_velocity : Inport  Port=3
  FK_info : Inport  Port=4
  joint_angle : Inport  Port=5
  joint_velocity : Inport  Port=6
  swing_state : Inport  Port=7
  hip_trajectory : Inport  Port=8
  knee_trajectory : Inport  Port=9
  Action Port : ActionPort  ActionType=case
  If Right stance / Left swing : If  IfExpression=u1 ==0
  Left Swing / Right Stance : Subsystem  TreatAsAtomicUnit=on
  Merge{1..5} (5 alike) : Merge
  Right Swing / Left Stance1 : Subsystem  TreatAsAtomicUnit=on
  Force : Outport
  Torques : Outport  Port=2
  r_vrp : Outport  Port=3
  r_extrapolated_CoM : Outport  Port=4
  Foot_adjust : Outport  Port=5
  wires:
  RorL/1 -> If Right stance / Left swing/1
  If Right stance / Left swing/1 -> Left Swing / Right Stance/Action
  If Right stance / Left swing/2 -> Right Swing / Left Stance1/Action
  Merge4/1 -> Force/1
  Merge1/1 -> Torques/1
  Merge2/1 -> r_vrp/1
  Merge3/1 -> r_extrapolated_CoM/1
  Left Swing / Right Stance/1(Force_des) -> Merge4/1
  Right Swing / Left Stance1/1(Force_des) -> Merge4/2
  Left Swing / Right Stance/2(Torques_des) -> Merge1/1
  Left Swing / Right Stance/3(r_vrp) -> Merge2/1
  Right Swing / Left Stance1/3(r_vrp) -> Merge2/2
  Left Swing / Right Stance/4(r_extrapolated_CoM) -> Merge3/1
  Right Swing / Left Stance1/4(r_extrapolated_CoM) -> Merge3/2
  DCM_position/1 -> Right Swing / Left Stance1/1(DCM_position), Left Swing / Right Stance/1(DCM_position)
  DCM_velocity/1 -> Right Swing / Left Stance1/2(DCM_velocity), Left Swing / Right Stance/2(DCM_velocity)
  FK_info/1 -> Right Swing / Left Stance1/3(FK_info), Left Swing / Right Stance/3(FK_info)
  joint_angle/1 -> Right Swing / Left Stance1/4(joint_angle), Left Swing / Right Stance/4(joint_angle)
  joint_velocity/1 -> Right Swing / Left Stance1/5(joint_velocity), Left Swing / Right Stance/5(joint_velocity)
  hip_trajectory/1 -> Right Swing / Left Stance1/7(hip_trajectory), Left Swing / Right Stance/7(hip_trajectory)
  swing_state/1 -> Right Swing / Left Stance1/6(swing_state), Left Swing / Right Stance/6(swing_state)
  Merge5/1 -> Foot_adjust/1
  Right Swing / Left Stance1/5(Foot_adjust) -> Merge5/2
  Left Swing / Right Stance/5(Foot_adjut) -> Merge5/1
  knee_trajectory/1 -> Right Swing / Left Stance1/8(knee_trajectory), Left Swing / Right Stance/8(knee_trajectory)
  Right Swing / Left Stance1/2(Torques_des) -> Merge1/2

== system Control_model_10DOF_fin/Control/Inititial_Transfert ==
  RorL : Inport
  DCM_position : Inport  Port=2
  DCM_velocity : Inport  Port=3
  FK_info : Inport  Port=4
  joint_angle : Inport  Port=5
  joint_velocity : Inport  Port=6
  hip_trajectory : Inport  Port=7
  Action Port : ActionPort  ActionType=case
  Constant : Constant  Value=0
  Constant2 : Constant  Value=[0;0;0]
  Demux : Demux  Outputs=3
  If Right stance phase : If  IfExpression=u1 ==0
  Left stance phase1 : Subsystem
  Merge{1..4} (4 alike) : Merge
  Mux : Mux  Inputs=3
  Right stance phase : Subsystem
  Terminator : Terminator
  Force : Outport
  Torques : Outport  Port=2
  r_vrp : Outport  Port=3
  r_extrapolated_CoM : Outport  Port=4
  Foot_adjust : Outport  Port=5
  wires:
  RorL/1 -> If Right stance phase/1
  If Right stance phase/1 -> Right stance phase/Action
  If Right stance phase/2 -> Left stance phase1/Action
  Merge1/1 -> Torques/1
  Merge2/1 -> r_vrp/1
  Merge3/1 -> r_extrapolated_CoM/1
  Right stance phase/1(Force_des) -> Merge4/1
  Left stance phase1/1(Force_des) -> Merge4/2
  Right stance phase/2(Torques_des) -> Merge1/1
  Left stance phase1/2(Torques_des) -> Merge1/2
  Right stance phase/3(r_vrp) -> Merge2/1
  Left stance phase1/3(r_vrp) -> Merge2/2
  Right stance phase/4(r_extrapolated_CoM) -> Merge3/1
  Left stance phase1/4(r_extrapolated_CoM) -> Merge3/2
  DCM_position/1 -> Left stance phase1/1(DCM_position), Right stance phase/1(DCM_position)
  DCM_velocity/1 -> Left stance phase1/2(DCM_velocity), Right stance phase/2(DCM_velocity)
  FK_info/1 -> Left stance phase1/3(FK_info), Right stance phase/3(FK_info)
  joint_angle/1 -> Left stance phase1/4(joint_angle), Right stance phase/4(joint_angle)
  joint_velocity/1 -> Left stance phase1/5(joint_velocity), Right stance phase/5(joint_velocity)
  hip_trajectory/1 -> Left stance phase1/6(hip_trajectory), Right stance phase/6(hip_trajectory)
  Constant2/1 -> Foot_adjust/1
  Demux/1 -> Mux/1
  Demux/2 -> Mux/2
  Merge4/1 -> Demux/1
  Mux/1 -> Force/1
  Constant/1 -> Mux/3
  Demux/3 -> Terminator/1

== system Control_model_10DOF_fin/Control/Single_Support ==
  RorL : Inport  OutDataTypeStr=boolean  PortDimensions=1
  DCM_position : Inport  Port=2
  DCM_velocity : Inport  Port=3
  FK_info : Inport  Port=4
  joint_angle : Inport  Port=5
  joint_velocity : Inport  Port=6
  swing_state : Inport  Port=7
  hip_trajectory : Inport  Port=8
  knee_trajectory : Inport  Port=9
  Action Port : ActionPort  ActionType=case
  If Right stance / Left swing : If  IfExpression=u1 ==0
  Left Swing / Right Stance : Subsystem  TreatAsAtomicUnit=on
  Merge{1..5} (5 alike) : Merge
  Right Swing / Left Stance : Subsystem  TreatAsAtomicUnit=on
  Force : Outport
  Torques : Outport  Port=2
  r_vrp : Outport  Port=3
  r_extrapolated_CoM : Outport  Port=4
  Foot_adjust : Outport  Port=5
  wires:
  RorL/1 -> If Right stance / Left swing/1
  If Right stance / Left swing/1 -> Left Swing / Right Stance/Action
  If Right stance / Left swing/2 -> Right Swing / Left Stance/Action
  Merge4/1 -> Force/1
  Merge1/1 -> Torques/1
  Merge2/1 -> r_vrp/1
  Merge3/1 -> r_extrapolated_CoM/1
  Left Swing / Right Stance/1(Force_des) -> Merge4/1
  Right Swing / Left Stance/1(Force_des) -> Merge4/2
  Left Swing / Right Stance/2(Torques_des) -> Merge1/1
  Right Swing / Left Stance/2(Torques_des) -> Merge1/2
  Left Swing / Right Stance/3(r_vrp) -> Merge2/1
  Right Swing / Left Stance/3(r_vrp) -> Merge2/2
  Left Swing / Right Stance/4(r_extrapolated_CoM) -> Merge3/1
  Right Swing / Left Stance/4(r_extrapolated_CoM) -> Merge3/2
  DCM_position/1 -> Right Swing / Left Stance/1(DCM_position), Left Swing / Right Stance/1(DCM_position)
  DCM_velocity/1 -> Left Swing / Right Stance/2(DCM_velocity), Right Swing / Left Stance/2(DCM_velocity)
  FK_info/1 -> Left Swing / Right Stance/3(FK_info), Right Swing / Left Stance/3(FK_info)
  joint_angle/1 -> Right Swing / Left Stance/4(joint_angle), Left Swing / Right Stance/4(joint_angle)
  joint_velocity/1 -> Right Swing / Left Stance/5(joint_velocity), Left Swing / Right Stance/5(joint_velocity)
  hip_trajectory/1 -> Right Swing / Left Stance/7(hip_trajectory), Left Swing / Right Stance/7(hip_trajectory)
  swing_state/1 -> Right Swing / Left Stance/6(swing_state), Left Swing / Right Stance/6(swing_state)
  Right Swing / Left Stance/5(Foot_adjust) -> Merge5/2
  Left Swing / Right Stance/5(Foot_adjust) -> Merge5/1
  Merge5/1 -> Foot_adjust/1
  knee_trajectory/1 -> Right Swing / Left Stance/8(knee_trajectory), Left Swing / Right Stance/8(knee_trajectory)

== system Control_model_10DOF_fin/Control/Stance_position ==
  angle : Inport
  velocity : Inport  Port=2
  Action Port : ActionPort  ActionType=case
  Constant{,1..3} (4 alike) : Constant  Value=[0;0;0]
  Stance control : Subsystem
  Force : Outport
  Torques : Outport  Port=2
  r_vrp : Outport  Port=3
  r_extrapolated_CoM : Outport  Port=4
  Foot_adjust : Outport  Port=5
  wires:
  angle/1 -> Stance control/1(angle)
  velocity/1 -> Stance control/2(velocity)
  Constant/1 -> Force/1
  Stance control/1(Torques) -> Torques/1
  Constant1/1 -> r_vrp/1
  Constant2/1 -> r_extrapolated_CoM/1
  Constant3/1 -> Foot_adjust/1

== system Control_model_10DOF_fin/Perturbation/Force ==
  Action Port : ActionPort
  Constant : Constant  Value=-280
  perturbation : Outport
  wires:
  Constant/1 -> perturbation/1

== system Control_model_10DOF_fin/Perturbation/Force1 ==
  Action Port : ActionPort
  Constant : Constant  Value=0
  perturbation : Outport
  wires:
  Constant/1 -> perturbation/1

== system Control_model_10DOF_fin/Time//State Machine/Hip_timer ==
  State : Inport
  time : Inport  Port=2
  RorL : Inport  Port=3
  Clock1 : Clock
  Clock2 : Clock
  DS : Subsystem  TreatAsAtomicUnit=on
  Finish_swing_phase : Subsystem  TreatAsAtomicUnit=on
  Initial_Transfert : Subsystem  TreatAsAtomicUnit=on
  Merge2 : Merge  Inputs=5
  SS : Subsystem  TreatAsAtomicUnit=on
  Sample and Hold : dspsigops/Sample and Hold  trig=Either edge  initCond=0  latchinput=on
  Stance_position : Subsystem  TreatAsAtomicUnit=on
  Sum1 : Sum  Inputs=|+-
  Switch Case : SwitchCase  CaseConditions={0,1,2,3,4}  ShowDefaultCase=off
  time_Hip : Outport
  wires:
  State/1 -> Switch Case/1
  Switch Case/1 -> Stance_position/Action
  Switch Case/2 -> Initial_Transfert/Action
  time/1 -> SS/1(time_swing), Initial_Transfert/1(time_DS)
  Switch Case/3 -> SS/Action
  Switch Case/4 -> Finish_swing_phase/Action
  Switch Case/5 -> DS/Action
  Stance_position/1(time_Hip) -> Merge2/1
  Initial_Transfert/1(time_Hip) -> Merge2/2
  SS/1(time_Hip) -> Merge2/3
  Finish_swing_phase/1(time_Hip) -> Merge2/4
  DS/1(time_Hip) -> Merge2/5
  Merge2/1 -> time_Hip/1
  Clock1/1 -> Sample and Hold/1
  Sample and Hold/1 -> Sum1/2
  Clock2/1 -> Sum1/1
  Sum1/1 -> DS/1(time)
  RorL/1 -> Sample and Hold/Trigger
